simulink model "building_EXAMPLE_v2_r2018b"  (R2018b)
settings: Solver=ode23tb  StartTime=-building.preruntime+8760*3600  StopTime=building.runtime+8760*3600  MaxStep=600  EnableMultiTasking=on
StartFcn:
  | tic
StopFcn:
  | toc
values from neighbouring files (symbols this model uses):
  building = building.add_simulation(1, 'Innsbruck - ERV, 120m3/h, 230 g/h', saveAIB, saveBDB, saveBOUNDARY, saveHVAC, 1)    [work_EXAMPLE_v1.m]
undefined symbols (not defined in the file or in its folder): cp, Dreifach, get_building, p, Qdot_C, Qdot_C_energy, Qdot_H, Qdot_H_energy, Qdot_I_electricity, Qdot_I_electricity_energy, Qdot_I_light, Qdot_I_light_energy, Qdot_I_person, Qdot_I_person_energy, Qdot_S, Qdot_S_energy, Qdot_T_ground, Qdot_T_ground_energy, Qdot_T_neighbour, Qdot_T_neighbour_energy, Qdot_T_opaque, Qdot_T_opaque_energy, Qdot_T_window, Qdot_T_window_energy, Qdot_V_infiltration, Qdot_V_infiltration_energy, Qdot_V_mech, Qdot_V_mech_energy, Qdot_V_window, Qdot_V_window_energy, rho, Tc, Tr, Ts, Wärmeschutzglas, x_CO2, x_H2O, x_VOC
libraries: carnotUIBK x1879, carnot x1
(part 8 of 28)

== system building_EXAMPLE_v2_r2018b/DATALOGGER/AIBz6 ==
  AIB : Inport
  AIB_initialize : carnotUIBK/room_node/EMPTY/AIB_initialize  SystemSampleTime=-1
  Bus Assignment1 : BusAssignment  AssignedSignals=Ts,Tc,Tr,x_H2O,x_CO2,x_VOC,rho,cp,p
  Bus Selector1 : BusSelector  OutputSignals=Ts,Tc,Tr,x_H2O,x_CO2,x_VOC,rho,cp,p
  AIB' : Outport
  wires:
  Bus Selector1/8 -> Bus Assignment1/9  "<cp>"
  Bus Selector1/7 -> Bus Assignment1/8  "<rho>"
  Bus Selector1/6 -> Bus Assignment1/7  "<x_VOC>"
  Bus Selector1/5 -> Bus Assignment1/6  "<x_CO2>"
  Bus Selector1/2 -> Bus Assignment1/3  "<Tc>"
  Bus Selector1/4 -> Bus Assignment1/5  "<x_H2O>"
  Bus Selector1/9 -> Bus Assignment1/10  "<p>"
  Bus Selector1/3 -> Bus Assignment1/4  "<Tr>"
  Bus Selector1/1 -> Bus Assignment1/2  "<Ts>"
  AIB_initialize/1 -> Bus Assignment1/1
  AIB/1 -> Bus Selector1/1
  Bus Assignment1/1 -> AIB'/1

== system building_EXAMPLE_v2_r2018b/DATALOGGER/AIBz7 ==
  AIB : Inport
  AIB_initialize : carnotUIBK/room_node/EMPTY/AIB_initialize  SystemSampleTime=-1
  Bus Assignment1 : BusAssignment  AssignedSignals=Ts,Tc,Tr,x_H2O,x_CO2,x_VOC,rho,cp,p
  Bus Selector1 : BusSelector  OutputSignals=Ts,Tc,Tr,x_H2O,x_CO2,x_VOC,rho,cp,p
  AIB' : Outport
  wires:
  Bus Assignment1/1 -> AIB'/1
  AIB/1 -> Bus Selector1/1
  AIB_initialize/1 -> Bus Assignment1/1
  Bus Selector1/1 -> Bus Assignment1/2  "<Ts>"
  Bus Selector1/3 -> Bus Assignment1/4  "<Tr>"
  Bus Selector1/9 -> Bus Assignment1/10  "<p>"
  Bus Selector1/4 -> Bus Assignment1/5  "<x_H2O>"
  Bus Selector1/2 -> Bus Assignment1/3  "<Tc>"
  Bus Selector1/5 -> Bus Assignment1/6  "<x_CO2>"
  Bus Selector1/6 -> Bus Assignment1/7  "<x_VOC>"
  Bus Selector1/7 -> Bus Assignment1/8  "<rho>"
  Bus Selector1/8 -> Bus Assignment1/9  "<cp>"

== system building_EXAMPLE_v2_r2018b/DATALOGGER/AIBz8 ==
  AIB : Inport
  AIB_initialize : carnotUIBK/room_node/EMPTY/AIB_initialize  SystemSampleTime=-1
  Bus Assignment1 : BusAssignment  AssignedSignals=Ts,Tc,Tr,x_H2O,x_CO2,x_VOC,rho,cp,p
  Bus Selector1 : BusSelector  OutputSignals=Ts,Tc,Tr,x_H2O,x_CO2,x_VOC,rho,cp,p
  AIB' : Outport
  wires:
  Bus Selector1/8 -> Bus Assignment1/9  "<cp>"
  Bus Selector1/7 -> Bus Assignment1/8  "<rho>"
  Bus Selector1/6 -> Bus Assignment1/7  "<x_VOC>"
  Bus Selector1/5 -> Bus Assignment1/6  "<x_CO2>"
  Bus Selector1/2 -> Bus Assignment1/3  "<Tc>"
  Bus Selector1/4 -> Bus Assignment1/5  "<x_H2O>"
  Bus Selector1/9 -> Bus Assignment1/10  "<p>"
  Bus Selector1/3 -> Bus Assignment1/4  "<Tr>"
  Bus Selector1/1 -> Bus Assignment1/2  "<Ts>"
  AIB_initialize/1 -> Bus Assignment1/1
  AIB/1 -> Bus Selector1/1
  Bus Assignment1/1 -> AIB'/1

== system building_EXAMPLE_v2_r2018b/DATALOGGER/AIBz9 ==
  AIB : Inport
  AIB_initialize : carnotUIBK/room_node/EMPTY/AIB_initialize  SystemSampleTime=-1
  Bus Assignment1 : BusAssignment  AssignedSignals=Ts,Tc,Tr,x_H2O,x_CO2,x_VOC,rho,cp,p
  Bus Selector1 : BusSelector  OutputSignals=Ts,Tc,Tr,x_H2O,x_CO2,x_VOC,rho,cp,p
  AIB' : Outport
  wires:
  Bus Assignment1/1 -> AIB'/1
  AIB/1 -> Bus Selector1/1
  AIB_initialize/1 -> Bus Assignment1/1
  Bus Selector1/1 -> Bus Assignment1/2  "<Ts>"
  Bus Selector1/3 -> Bus Assignment1/4  "<Tr>"
  Bus Selector1/9 -> Bus Assignment1/10  "<p>"
  Bus Selector1/4 -> Bus Assignment1/5  "<x_H2O>"
  Bus Selector1/2 -> Bus Assignment1/3  "<Tc>"
  Bus Selector1/5 -> Bus Assignment1/6  "<x_CO2>"
  Bus Selector1/6 -> Bus Assignment1/7  "<x_VOC>"
  Bus Selector1/7 -> Bus Assignment1/8  "<rho>"
  Bus Selector1/8 -> Bus Assignment1/9  "<cp>"

== system building_EXAMPLE_v2_r2018b/DATALOGGER/logger_AIB ==
  AIB : Inport
  Enable : EnablePort
  saveAIB : ToWorkspace  VariableName=saveAIB  SaveFormat=Timeseries  SampleTime=building.get_building().sampletime_1
  wires:
  AIB/1 -> saveAIB/1

== system building_EXAMPLE_v2_r2018b/DATALOGGER/logger_BDB ==
  note: CHANGE BDB TO THE CORRESPONDING ZONE!!!!
  BDB : Inport
  Enable : EnablePort
  Bus Creator : BusCreator  Inputs=2
  Bus Creator1 : BusCreator  Inputs=10
  saveBDB : ToWorkspace  VariableName=saveBDB  SaveFormat=Timeseries  SampleTime=building.get_building().sampletime_1
  z1 : Subsystem
  z10 : Subsystem
  z2 : Subsystem
  z3 : Subsystem
  z4 : Subsystem
  z5 : Subsystem
  z6 : Subsystem
  z7 : Subsystem
  z8 : Subsystem
  z9 : Subsystem
  wires:
  BDB/1 -> Bus Creator/1, z1/1(BDB), z2/1(BDB), z3/1(BDB), z4/1(BDB), z5/1(BDB), z6/1(BDB), z7/1(BDB), z8/1(BDB), z10/1(BDB), z9/1(BDB)  "power"
  Bus Creator/1 -> saveBDB/1
  z1/1(BDBenergy) -> Bus Creator1/1  "z1"
  z4/1(BDBenergy) -> Bus Creator1/4  "z4"
  z3/1(BDBenergy) -> Bus Creator1/3  "z3"
  z2/1(BDBenergy) -> Bus Creator1/2  "z2"
  z10/1(BDBenergy) -> Bus Creator1/10  "z10"
  z9/1(BDBenergy) -> Bus Creator1/9  "z9"
  z8/1(BDBenergy) -> Bus Creator1/8  "z8"
  z7/1(BDBenergy) -> Bus Creator1/7  "z7"
  z6/1(BDBenergy) -> Bus Creator1/6  "z6"
  z5/1(BDBenergy) -> Bus Creator1/5  "z5"
  Bus Creator1/1 -> Bus Creator/2  "energy"

== system building_EXAMPLE_v2_r2018b/DATALOGGER/logger_BOUNDARY ==
  BOUNDARY : Inport
  Enable : EnablePort
  Bus Creator : BusCreator  Inputs=2
  Bus Creator1 : BusCreator  Inputs=4
  Bus Selector : BusSelector  OutputSignals=WDB.Solar_Radiation_beam_normal,WDB.Solar_Radiation_diffuse_horizontal,WDB.Solar_Radiation_direct_surface,WDB.Solar_Radiation_diffuse_surface  OutputAsBus=on
  Demux : Demux
  Integrator : Integrator
  Ws->kWh : Gain  Gain=1/3600/1000
  saveBOUNDARY : ToWorkspace  VariableName=saveBOUNDARY  SaveFormat=Timeseries  SampleTime=building.get_building().sampletime_1
  wires:
  BOUNDARY/1 -> Bus Selector/1, Bus Creator/1  "power"
  Bus Creator/1 -> saveBOUNDARY/1
  Bus Selector/1 -> Integrator/1
  Integrator/1 -> Ws->kWh/1
  Demux/1 -> Bus Creator1/1  "Solar_Radiation_beam_normal_Energy"
  Demux/2 -> Bus Creator1/2  "Solar_Radiation_diffuse_horizontal_Energy"
  Demux/4 -> Bus Creator1/4  "Solar_Radiation_diffuse_surface_Energy"
  Demux/3 -> Bus Creator1/3  "Solar_Radiation_direct_surface_Energy"
  Bus Creator1/1 -> Bus Creator/2  "energy"
  Ws->kWh/1 -> Demux/1

== system building_EXAMPLE_v2_r2018b/DATALOGGER/logger_HVAC ==
  HVAC : Inport
  Enable : EnablePort
  saveHVAC : ToWorkspace  VariableName=saveHVAC  SaveFormat=Timeseries  SampleTime=building.get_building().sampletime_1
  wires:
  HVAC/1 -> saveHVAC/1

== system building_EXAMPLE_v2_r2018b/DATALOGGER/z1 ==
  BDB : Inport
  BDB_initialize : carnotUIBK/room_node/EMPTY/BDB_initialize  SystemSampleTime=-1
  Bus Assignment : BusAssignment  AssignedSignals=Qdot_T_opaque,Qdot_T_ground,Qdot_T_neighbour,Qdot_T_window,Qdot_V_mech,Qdot_V_window,Qdot_V_infiltration,Qdot_S,Qdot_I_person,Qdot_I_light,Qdot_I_electricity,Qdot_H,Qdot_C
  Bus Selector1 : BusSelector  OutputSignals=Qdot_T_opaque,Qdot_T_ground,Qdot_T_neighbour,Qdot_T_window,Qdot_V_mech,Qdot_V_window,Qdot_V_infiltration,Qdot_S,Qdot_I_person,Qdot_I_light,Qdot_I_electricity,Qdot_H,Qdot_C
  BDB' : Outport
  wires:
  BDB/1 -> Bus Selector1/1
  Bus Assignment/1 -> BDB'/1
  BDB_initialize/1 -> Bus Assignment/1
  Bus Selector1/1 -> Bus Assignment/2  "<Qdot_T_opaque>"
  Bus Selector1/13 -> Bus Assignment/14  "<Qdot_C>"
  Bus Selector1/12 -> Bus Assignment/13  "<Qdot_H>"
  Bus Selector1/11 -> Bus Assignment/12  "<Qdot_I_electricity>"
  Bus Selector1/10 -> Bus Assignment/11  "<Qdot_I_light>"
  Bus Selector1/9 -> Bus Assignment/10  "<Qdot_I_person>"
  Bus Selector1/8 -> Bus Assignment/9  "<Qdot_S>"
  Bus Selector1/7 -> Bus Assignment/8  "<Qdot_V_infiltration>"
  Bus Selector1/6 -> Bus Assignment/7  "<Qdot_V_window>"
  Bus Selector1/5 -> Bus Assignment/6  "<Qdot_V_mech>"
  Bus Selector1/4 -> Bus Assignment/5  "<Qdot_T_window>"
  Bus Selector1/3 -> Bus Assignment/4  "<Qdot_T_neighbour>"
  Bus Selector1/2 -> Bus Assignment/3  "<Qdot_T_ground>"

== system building_EXAMPLE_v2_r2018b/DATALOGGER/z10 ==
  BDB : Inport
  BDB_initialize : carnotUIBK/room_node/EMPTY/BDB_initialize  SystemSampleTime=-1
  Bus Assignment : BusAssignment  AssignedSignals=Qdot_T_opaque,Qdot_T_ground,Qdot_T_neighbour,Qdot_T_window,Qdot_V_mech,Qdot_V_window,Qdot_V_infiltration,Qdot_S,Qdot_I_person,Qdot_I_light,Qdot_I_electricity,Qdot_H,Qdot_C
  Bus Selector1 : BusSelector  OutputSignals=Qdot_T_opaque,Qdot_T_ground,Qdot_T_neighbour,Qdot_T_window,Qdot_V_mech,Qdot_V_window,Qdot_V_infiltration,Qdot_S,Qdot_I_person,Qdot_I_light,Qdot_I_electricity,Qdot_H,Qdot_C
  BDB' : Outport
  wires:
  Bus Selector1/2 -> Bus Assignment/3  "<Qdot_T_ground>"
  Bus Selector1/3 -> Bus Assignment/4  "<Qdot_T_neighbour>"
  Bus Selector1/4 -> Bus Assignment/5  "<Qdot_T_window>"
  Bus Selector1/5 -> Bus Assignment/6  "<Qdot_V_mech>"
  Bus Selector1/6 -> Bus Assignment/7  "<Qdot_V_window>"
  Bus Selector1/7 -> Bus Assignment/8  "<Qdot_V_infiltration>"
  Bus Selector1/8 -> Bus Assignment/9  "<Qdot_S>"
  Bus Selector1/9 -> Bus Assignment/10  "<Qdot_I_person>"
  Bus Selector1/10 -> Bus Assignment/11  "<Qdot_I_light>"
  Bus Selector1/11 -> Bus Assignment/12  "<Qdot_I_electricity>"
  Bus Selector1/12 -> Bus Assignment/13  "<Qdot_H>"
  Bus Selector1/13 -> Bus Assignment/14  "<Qdot_C>"
  Bus Selector1/1 -> Bus Assignment/2  "<Qdot_T_opaque>"
  BDB_initialize/1 -> Bus Assignment/1
  Bus Assignment/1 -> BDB'/1
  BDB/1 -> Bus Selector1/1

== system building_EXAMPLE_v2_r2018b/DATALOGGER/z2 ==
  BDB : Inport
  BDB_initialize : carnotUIBK/room_node/EMPTY/BDB_initialize  SystemSampleTime=-1
  Bus Assignment : BusAssignment  AssignedSignals=Qdot_T_opaque,Qdot_T_ground,Qdot_T_neighbour,Qdot_T_window,Qdot_V_mech,Qdot_V_window,Qdot_V_infiltration,Qdot_S,Qdot_I_person,Qdot_I_light,Qdot_I_electricity,Qdot_H,Qdot_C
  Bus Selector1 : BusSelector  OutputSignals=Qdot_T_opaque,Qdot_T_ground,Qdot_T_neighbour,Qdot_T_window,Qdot_V_mech,Qdot_V_window,Qdot_V_infiltration,Qdot_S,Qdot_I_person,Qdot_I_light,Qdot_I_electricity,Qdot_H,Qdot_C
  BDB' : Outport
  wires:
  Bus Selector1/2 -> Bus Assignment/3  "<Qdot_T_ground>"
  Bus Selector1/3 -> Bus Assignment/4  "<Qdot_T_neighbour>"
  Bus Selector1/4 -> Bus Assignment/5  "<Qdot_T_window>"
  Bus Selector1/5 -> Bus Assignment/6  "<Qdot_V_mech>"
  Bus Selector1/6 -> Bus Assignment/7  "<Qdot_V_window>"
  Bus Selector1/7 -> Bus Assignment/8  "<Qdot_V_infiltration>"
  Bus Selector1/8 -> Bus Assignment/9  "<Qdot_S>"
  Bus Selector1/9 -> Bus Assignment/10  "<Qdot_I_person>"
  Bus Selector1/10 -> Bus Assignment/11  "<Qdot_I_light>"
  Bus Selector1/11 -> Bus Assignment/12  "<Qdot_I_electricity>"
  Bus Selector1/12 -> Bus Assignment/13  "<Qdot_H>"
  Bus Selector1/13 -> Bus Assignment/14  "<Qdot_C>"
  Bus Selector1/1 -> Bus Assignment/2  "<Qdot_T_opaque>"
  BDB_initialize/1 -> Bus Assignment/1
  Bus Assignment/1 -> BDB'/1
  BDB/1 -> Bus Selector1/1

== system building_EXAMPLE_v2_r2018b/DATALOGGER/z3 ==
  BDB : Inport
  BDB_initialize : carnotUIBK/room_node/EMPTY/BDB_initialize  SystemSampleTime=-1
  Bus Assignment : BusAssignment  AssignedSignals=Qdot_T_opaque,Qdot_T_ground,Qdot_T_neighbour,Qdot_T_window,Qdot_V_mech,Qdot_V_window,Qdot_V_infiltration,Qdot_S,Qdot_I_person,Qdot_I_light,Qdot_I_electricity,Qdot_H,Qdot_C
  Bus Selector1 : BusSelector  OutputSignals=Qdot_T_opaque,Qdot_T_ground,Qdot_T_neighbour,Qdot_T_window,Qdot_V_mech,Qdot_V_window,Qdot_V_infiltration,Qdot_S,Qdot_I_person,Qdot_I_light,Qdot_I_electricity,Qdot_H,Qdot_C
  BDB' : Outport
  wires:
  BDB/1 -> Bus Selector1/1
  Bus Assignment/1 -> BDB'/1
  BDB_initialize/1 -> Bus Assignment/1
  Bus Selector1/1 -> Bus Assignment/2  "<Qdot_T_opaque>"
  Bus Selector1/13 -> Bus Assignment/14  "<Qdot_C>"
  Bus Selector1/12 -> Bus Assignment/13  "<Qdot_H>"
  Bus Selector1/11 -> Bus Assignment/12  "<Qdot_I_electricity>"
  Bus Selector1/10 -> Bus Assignment/11  "<Qdot_I_light>"
  Bus Selector1/9 -> Bus Assignment/10  "<Qdot_I_person>"
  Bus Selector1/8 -> Bus Assignment/9  "<Qdot_S>"
  Bus Selector1/7 -> Bus Assignment/8  "<Qdot_V_infiltration>"
  Bus Selector1/6 -> Bus Assignment/7  "<Qdot_V_window>"
  Bus Selector1/5 -> Bus Assignment/6  "<Qdot_V_mech>"
  Bus Selector1/4 -> Bus Assignment/5  "<Qdot_T_window>"
  Bus Selector1/3 -> Bus Assignment/4  "<Qdot_T_neighbour>"
  Bus Selector1/2 -> Bus Assignment/3  "<Qdot_T_ground>"

== system building_EXAMPLE_v2_r2018b/DATALOGGER/z4 ==
  BDB : Inport
  BDB_initialize : carnotUIBK/room_node/EMPTY/BDB_initialize  SystemSampleTime=-1
  Bus Assignment : BusAssignment  AssignedSignals=Qdot_T_opaque,Qdot_T_ground,Qdot_T_neighbour,Qdot_T_window,Qdot_V_mech,Qdot_V_window,Qdot_V_infiltration,Qdot_S,Qdot_I_person,Qdot_I_light,Qdot_I_electricity,Qdot_H,Qdot_C
  Bus Selector1 : BusSelector  OutputSignals=Qdot_T_opaque,Qdot_T_ground,Qdot_T_neighbour,Qdot_T_window,Qdot_V_mech,Qdot_V_window,Qdot_V_infiltration,Qdot_S,Qdot_I_person,Qdot_I_light,Qdot_I_electricity,Qdot_H,Qdot_C
  BDB' : Outport
  wires:
  Bus Selector1/2 -> Bus Assignment/3  "<Qdot_T_ground>"
  Bus Selector1/3 -> Bus Assignment/4  "<Qdot_T_neighbour>"
  Bus Selector1/4 -> Bus Assignment/5  "<Qdot_T_window>"
  Bus Selector1/5 -> Bus Assignment/6  "<Qdot_V_mech>"
  Bus Selector1/6 -> Bus Assignment/7  "<Qdot_V_window>"
  Bus Selector1/7 -> Bus Assignment/8  "<Qdot_V_infiltration>"
  Bus Selector1/8 -> Bus Assignment/9  "<Qdot_S>"
  Bus Selector1/9 -> Bus Assignment/10  "<Qdot_I_person>"
  Bus Selector1/10 -> Bus Assignment/11  "<Qdot_I_light>"
  Bus Selector1/11 -> Bus Assignment/12  "<Qdot_I_electricity>"
  Bus Selector1/12 -> Bus Assignment/13  "<Qdot_H>"
  Bus Selector1/13 -> Bus Assignment/14  "<Qdot_C>"
  Bus Selector1/1 -> Bus Assignment/2  "<Qdot_T_opaque>"
  BDB_initialize/1 -> Bus Assignment/1
  Bus Assignment/1 -> BDB'/1
  BDB/1 -> Bus Selector1/1

== system building_EXAMPLE_v2_r2018b/DATALOGGER/z5 ==
  BDB : Inport
  BDB_initialize : carnotUIBK/room_node/EMPTY/BDB_initialize  SystemSampleTime=-1
  Bus Assignment : BusAssignment  AssignedSignals=Qdot_T_opaque,Qdot_T_ground,Qdot_T_neighbour,Qdot_T_window,Qdot_V_mech,Qdot_V_window,Qdot_V_infiltration,Qdot_S,Qdot_I_person,Qdot_I_light,Qdot_I_electricity,Qdot_H,Qdot_C
  Bus Selector1 : BusSelector  OutputSignals=Qdot_T_opaque,Qdot_T_ground,Qdot_T_neighbour,Qdot_T_window,Qdot_V_mech,Qdot_V_window,Qdot_V_infiltration,Qdot_S,Qdot_I_person,Qdot_I_light,Qdot_I_electricity,Qdot_H,Qdot_C
  BDB' : Outport
  wires:
  BDB/1 -> Bus Selector1/1
  Bus Assignment/1 -> BDB'/1
  BDB_initialize/1 -> Bus Assignment/1
  Bus Selector1/1 -> Bus Assignment/2  "<Qdot_T_opaque>"
  Bus Selector1/13 -> Bus Assignment/14  "<Qdot_C>"
  Bus Selector1/12 -> Bus Assignment/13  "<Qdot_H>"
  Bus Selector1/11 -> Bus Assignment/12  "<Qdot_I_electricity>"
  Bus Selector1/10 -> Bus Assignment/11  "<Qdot_I_light>"
  Bus Selector1/9 -> Bus Assignment/10  "<Qdot_I_person>"
  Bus Selector1/8 -> Bus Assignment/9  "<Qdot_S>"
  Bus Selector1/7 -> Bus Assignment/8  "<Qdot_V_infiltration>"
  Bus Selector1/6 -> Bus Assignment/7  "<Qdot_V_window>"
  Bus Selector1/5 -> Bus Assignment/6  "<Qdot_V_mech>"
  Bus Selector1/4 -> Bus Assignment/5  "<Qdot_T_window>"
  Bus Selector1/3 -> Bus Assignment/4  "<Qdot_T_neighbour>"
  Bus Selector1/2 -> Bus Assignment/3  "<Qdot_T_ground>"

== system building_EXAMPLE_v2_r2018b/DATALOGGER/z6 ==
  BDB : Inport
  BDB_initialize : carnotUIBK/room_node/EMPTY/BDB_initialize  SystemSampleTime=-1
  Bus Assignment : BusAssignment  AssignedSignals=Qdot_T_opaque,Qdot_T_ground,Qdot_T_neighbour,Qdot_T_window,Qdot_V_mech,Qdot_V_window,Qdot_V_infiltration,Qdot_S,Qdot_I_person,Qdot_I_light,Qdot_I_electricity,Qdot_H,Qdot_C
  Bus Selector1 : BusSelector  OutputSignals=Qdot_T_opaque,Qdot_T_ground,Qdot_T_neighbour,Qdot_T_window,Qdot_V_mech,Qdot_V_window,Qdot_V_infiltration,Qdot_S,Qdot_I_person,Qdot_I_light,Qdot_I_electricity,Qdot_H,Qdot_C
  BDB' : Outport
  wires:
  Bus Selector1/2 -> Bus Assignment/3  "<Qdot_T_ground>"
  Bus Selector1/3 -> Bus Assignment/4  "<Qdot_T_neighbour>"
  Bus Selector1/4 -> Bus Assignment/5  "<Qdot_T_window>"
  Bus Selector1/5 -> Bus Assignment/6  "<Qdot_V_mech>"
  Bus Selector1/6 -> Bus Assignment/7  "<Qdot_V_window>"
  Bus Selector1/7 -> Bus Assignment/8  "<Qdot_V_infiltration>"
  Bus Selector1/8 -> Bus Assignment/9  "<Qdot_S>"
  Bus Selector1/9 -> Bus Assignment/10  "<Qdot_I_person>"
  Bus Selector1/10 -> Bus Assignment/11  "<Qdot_I_light>"
  Bus Selector1/11 -> Bus Assignment/12  "<Qdot_I_electricity>"
  Bus Selector1/12 -> Bus Assignment/13  "<Qdot_H>"
  Bus Selector1/13 -> Bus Assignment/14  "<Qdot_C>"
  Bus Selector1/1 -> Bus Assignment/2  "<Qdot_T_opaque>"
  BDB_initialize/1 -> Bus Assignment/1
  Bus Assignment/1 -> BDB'/1
  BDB/1 -> Bus Selector1/1

== system building_EXAMPLE_v2_r2018b/DATALOGGER/z7 ==
  BDB : Inport
  BDB_initialize : carnotUIBK/room_node/EMPTY/BDB_initialize  SystemSampleTime=-1
  Bus Assignment : BusAssignment  AssignedSignals=Qdot_T_opaque,Qdot_T_ground,Qdot_T_neighbour,Qdot_T_window,Qdot_V_mech,Qdot_V_window,Qdot_V_infiltration,Qdot_S,Qdot_I_person,Qdot_I_light,Qdot_I_electricity,Qdot_H,Qdot_C
  Bus Selector1 : BusSelector  OutputSignals=Qdot_T_opaque,Qdot_T_ground,Qdot_T_neighbour,Qdot_T_window,Qdot_V_mech,Qdot_V_window,Qdot_V_infiltration,Qdot_S,Qdot_I_person,Qdot_I_light,Qdot_I_electricity,Qdot_H,Qdot_C
  BDB' : Outport
  wires:
  BDB/1 -> Bus Selector1/1
  Bus Assignment/1 -> BDB'/1
  BDB_initialize/1 -> Bus Assignment/1
  Bus Selector1/1 -> Bus Assignment/2  "<Qdot_T_opaque>"
  Bus Selector1/13 -> Bus Assignment/14  "<Qdot_C>"
  Bus Selector1/12 -> Bus Assignment/13  "<Qdot_H>"
  Bus Selector1/11 -> Bus Assignment/12  "<Qdot_I_electricity>"
  Bus Selector1/10 -> Bus Assignment/11  "<Qdot_I_light>"
  Bus Selector1/9 -> Bus Assignment/10  "<Qdot_I_person>"
  Bus Selector1/8 -> Bus Assignment/9  "<Qdot_S>"
  Bus Selector1/7 -> Bus Assignment/8  "<Qdot_V_infiltration>"
  Bus Selector1/6 -> Bus Assignment/7  "<Qdot_V_window>"
  Bus Selector1/5 -> Bus Assignment/6  "<Qdot_V_mech>"
  Bus Selector1/4 -> Bus Assignment/5  "<Qdot_T_window>"
  Bus Selector1/3 -> Bus Assignment/4  "<Qdot_T_neighbour>"
  Bus Selector1/2 -> Bus Assignment/3  "<Qdot_T_ground>"

== system building_EXAMPLE_v2_r2018b/DATALOGGER/z8 ==
  BDB : Inport
  BDB_initialize : carnotUIBK/room_node/EMPTY/BDB_initialize  SystemSampleTime=-1
  Bus Assignment : BusAssignment  AssignedSignals=Qdot_T_opaque,Qdot_T_ground,Qdot_T_neighbour,Qdot_T_window,Qdot_V_mech,Qdot_V_window,Qdot_V_infiltration,Qdot_S,Qdot_I_person,Qdot_I_light,Qdot_I_electricity,Qdot_H,Qdot_C
  Bus Selector1 : BusSelector  OutputSignals=Qdot_T_opaque,Qdot_T_ground,Qdot_T_neighbour,Qdot_T_window,Qdot_V_mech,Qdot_V_window,Qdot_V_infiltration,Qdot_S,Qdot_I_person,Qdot_I_light,Qdot_I_electricity,Qdot_H,Qdot_C
  BDB' : Outport
  wires:
  Bus Selector1/2 -> Bus Assignment/3  "<Qdot_T_ground>"
  Bus Selector1/3 -> Bus Assignment/4  "<Qdot_T_neighbour>"
  Bus Selector1/4 -> Bus Assignment/5  "<Qdot_T_window>"
  Bus Selector1/5 -> Bus Assignment/6  "<Qdot_V_mech>"
  Bus Selector1/6 -> Bus Assignment/7  "<Qdot_V_window>"
  Bus Selector1/7 -> Bus Assignment/8  "<Qdot_V_infiltration>"
  Bus Selector1/8 -> Bus Assignment/9  "<Qdot_S>"
  Bus Selector1/9 -> Bus Assignment/10  "<Qdot_I_person>"
  Bus Selector1/10 -> Bus Assignment/11  "<Qdot_I_light>"
  Bus Selector1/11 -> Bus Assignment/12  "<Qdot_I_electricity>"
  Bus Selector1/12 -> Bus Assignment/13  "<Qdot_H>"
  Bus Selector1/13 -> Bus Assignment/14  "<Qdot_C>"
  Bus Selector1/1 -> Bus Assignment/2  "<Qdot_T_opaque>"
  BDB_initialize/1 -> Bus Assignment/1
  Bus Assignment/1 -> BDB'/1
  BDB/1 -> Bus Selector1/1

== system building_EXAMPLE_v2_r2018b/DATALOGGER/z9 ==
  BDB : Inport
  BDB_initialize : carnotUIBK/room_node/EMPTY/BDB_initialize  SystemSampleTime=-1
  Bus Assignment : BusAssignment  AssignedSignals=Qdot_T_opaque,Qdot_T_ground,Qdot_T_neighbour,Qdot_T_window,Qdot_V_mech,Qdot_V_window,Qdot_V_infiltration,Qdot_S,Qdot_I_person,Qdot_I_light,Qdot_I_electricity,Qdot_H,Qdot_C
  Bus Selector1 : BusSelector  OutputSignals=Qdot_T_opaque,Qdot_T_ground,Qdot_T_neighbour,Qdot_T_window,Qdot_V_mech,Qdot_V_window,Qdot_V_infiltration,Qdot_S,Qdot_I_person,Qdot_I_light,Qdot_I_electricity,Qdot_H,Qdot_C
  BDB' : Outport
  wires:
  BDB/1 -> Bus Selector1/1
  Bus Assignment/1 -> BDB'/1
  BDB_initialize/1 -> Bus Assignment/1
  Bus Selector1/1 -> Bus Assignment/2  "<Qdot_T_opaque>"
  Bus Selector1/13 -> Bus Assignment/14  "<Qdot_C>"
  Bus Selector1/12 -> Bus Assignment/13  "<Qdot_H>"
  Bus Selector1/11 -> Bus Assignment/12  "<Qdot_I_electricity>"
  Bus Selector1/10 -> Bus Assignment/11  "<Qdot_I_light>"
  Bus Selector1/9 -> Bus Assignment/10  "<Qdot_I_person>"
  Bus Selector1/8 -> Bus Assignment/9  "<Qdot_S>"
  Bus Selector1/7 -> Bus Assignment/8  "<Qdot_V_infiltration>"
  Bus Selector1/6 -> Bus Assignment/7  "<Qdot_V_window>"
  Bus Selector1/5 -> Bus Assignment/6  "<Qdot_V_mech>"
  Bus Selector1/4 -> Bus Assignment/5  "<Qdot_T_window>"
  Bus Selector1/3 -> Bus Assignment/4  "<Qdot_T_neighbour>"
  Bus Selector1/2 -> Bus Assignment/3  "<Qdot_T_ground>"

== system building_EXAMPLE_v2_r2018b/BUILDING/INTERSECTION_1_10/airexchange_1 ==
  AIB1 : Inport
  AIB2 : Inport  Port=2
  control : Inport  Port=3
  EMPTY : carnotUIBK/airexchange_intersection/EMPTY  VariantControl=(default)
  airexchange_empiric : carnotUIBK/airexchange_intersection/airexchange_empiric  VariantControl=V_i_1_10_inf1_m0
  airexchange_powerlaw : carnotUIBK/airexchange_intersection/airexchange_powerlaw  VariantControl=V_i_1_10_inf1_m1
  "[S1]" : Outport
  "[S2]" : Outport  Port=2

== system building_EXAMPLE_v2_r2018b/BUILDING/INTERSECTION_1_10/airexchange_2 ==
  AIB1 : Inport
  AIB2 : Inport  Port=2
  control : Inport  Port=3
  EMPTY : carnotUIBK/airexchange_intersection/EMPTY  VariantControl=(default)
  airexchange_empiric : carnotUIBK/airexchange_intersection/airexchange_empiric  VariantControl=V_i_1_10_inf2_m0
  airexchange_powerlaw : carnotUIBK/airexchange_intersection/airexchange_powerlaw  VariantControl=V_i_1_10_inf2_m1
  "[S1]" : Outport
  "[S2]" : Outport  Port=2

== system building_EXAMPLE_v2_r2018b/BUILDING/INTERSECTION_1_10/airexchange_3 ==
  AIB1 : Inport
  AIB2 : Inport  Port=2
  control : Inport  Port=3
  EMPTY : carnotUIBK/airexchange_intersection/EMPTY  VariantControl=(default)
  airexchange_empiric : carnotUIBK/airexchange_intersection/airexchange_empiric  VariantControl=V_i_1_10_inf3_m0
  airexchange_powerlaw : carnotUIBK/airexchange_intersection/airexchange_powerlaw  VariantControl=V_i_1_10_inf3_m1
  "[S1]" : Outport
  "[S2]" : Outport  Port=2

== system building_EXAMPLE_v2_r2018b/BUILDING/INTERSECTION_1_10/wall_1 ==
  AIB1 : Inport
  AIB2 : Inport  Port=2
  Qdot_sol1 : Inport  Port=3
  Qdot_sol2 : Inport  Port=4
  EMPTY : carnotUIBK/wall_intersection/EMPTY  VariantControl=(default)
  R-C model : carnotUIBK/wall_intersection/R-C model  VariantControl=V_i_1_10_w1_m1  t0=z.t_ini  d=fliplr(const.parameter.xmesh_beu)  cond=fliplr(const.parameter.lambda)  cwall=fliplr(const.parameter.cp)  rho=fliplr(const.parameter.rho)  reflectground=0.2  abs_emiss=[const.absorption_2 const.emission_2 const.emission_1]  tau=const.parameter.tau  dactive=const.parameter.d_active
      link override alpha_i1/alpha_i_down: VariantControl=V_i_1_10_w1_hti2
      link override alpha_i1/alpha_i_horizontal: VariantControl=V_i_1_10_w1_hti0
      link override alpha_i1/alpha_i_up: VariantControl=V_i_1_10_w1_hti1
      link override alpha_i2/alpha_i_down: VariantControl=V_i_1_10_w1_hti2
      link override alpha_i2/alpha_i_horizontal: VariantControl=V_i_1_10_w1_hti0
      link override alpha_i2/alpha_i_up: VariantControl=V_i_1_10_w1_hti1
  UA : carnotUIBK/wall_intersection/UA  VariantControl=V_i_1_10_w1_m0  U=const.parameter.U
      link override Rsi/down: VariantControl=V_i_1_10_w1_hti2
      link override Rsi/horizontal: VariantControl=V_i_1_10_w1_hti0
      link override Rsi/up: VariantControl=V_i_1_10_w1_hti1
  hygrothermal model : carnotUIBK/wall_intersection/hygrothermal model  VariantControl=V_i_1_10_w1_m2  t0=z.t_ini  reflectground=0.2  abs_emiss=[const.absorption_2 const.emission_2 const.emission_1]  xmesh=const.parameter.xmesh_hygro  X=const.parameter.X  d=const.parameter.d  lambda=const.parameter.lambda_hygro  rho=const.parameter.rho_hygro  cp=const.parameter.cp_hygro  mu=const.parameter.mu  ufs=const.parameter.ufs  FSF_u=const.parameter.FSF_u  FSF_phi=const.parameter.FSF_phi  FSF_dudphi=const.parameter.FSF_dudphi  FSF_k=const.parameter.FSF_k  K_kleff=const.parameter.K_kleff  K_u=const.parameter.K_u  K_kl=const.parameter.K_kl  FSF_length=const.parameter.FSF_length  K_length=const.parameter.K_length  T_ini=const.parameter.T_ini_hygro  Phi_ini=const.parameter.Phi_ini_hygro  T_source=const.parameter.T_source  Phi_source=const.parameter.Phi_source  Tdactive=const.parameter.T_dactive  Phidactive=const.parameter.Phi_dactive
      link override alpha_i1/alpha_i_down: VariantControl=V_i_1_10_w1_hti2
      link override alpha_i1/alpha_i_horizontal: VariantControl=V_i_1_10_w1_hti0
      link override alpha_i1/alpha_i_up: VariantControl=V_i_1_10_w1_hti1
      link override alpha_i2/alpha_i_down: VariantControl=V_i_1_10_w1_hti2
      link override alpha_i2/alpha_i_horizontal: VariantControl=V_i_1_10_w1_hti0
      link override alpha_i2/alpha_i_up: VariantControl=V_i_1_10_w1_hti1
  "[S1]" : Outport
  "[S2]" : Outport  Port=2

== system building_EXAMPLE_v2_r2018b/BUILDING/INTERSECTION_1_10/wall_2 ==
  AIB1 : Inport
  AIB2 : Inport  Port=2
  Qdot_sol1 : Inport  Port=3
  Qdot_sol2 : Inport  Port=4
  EMPTY : carnotUIBK/wall_intersection/EMPTY  VariantControl=(default)
  R-C model : carnotUIBK/wall_intersection/R-C model  VariantControl=V_i_1_10_w2_m1  t0=z.t_ini  d=fliplr(const.parameter.xmesh_beu)  cond=fliplr(const.parameter.lambda)  cwall=fliplr(const.parameter.cp)  rho=fliplr(const.parameter.rho)  reflectground=0.2  abs_emiss=[const.absorption_2 const.emission_2 const.emission_1]  tau=const.parameter.tau  dactive=const.parameter.d_active
      link override alpha_i1/alpha_i_down: VariantControl=V_i_1_10_w2_hti2
      link override alpha_i1/alpha_i_horizontal: VariantControl=V_i_1_10_w2_hti0
      link override alpha_i1/alpha_i_up: VariantControl=V_i_1_10_w2_hti1
      link override alpha_i2/alpha_i_down: VariantControl=V_i_1_10_w2_hti2
      link override alpha_i2/alpha_i_horizontal: VariantControl=V_i_1_10_w2_hti0
      link override alpha_i2/alpha_i_up: VariantControl=V_i_1_10_w2_hti1
  UA : carnotUIBK/wall_intersection/UA  VariantControl=V_i_1_10_w2_m0  U=const.parameter.U
      link override Rsi/down: VariantControl=V_i_1_10_w2_hti2
      link override Rsi/horizontal: VariantControl=V_i_1_10_w2_hti0
      link override Rsi/up: VariantControl=V_i_1_10_w2_hti1
  hygrothermal model : carnotUIBK/wall_intersection/hygrothermal model  VariantControl=V_i_1_10_w2_m2  t0=z.t_ini  reflectground=0.2  abs_emiss=[const.absorption_2 const.emission_2 const.emission_1]  xmesh=const.parameter.xmesh_hygro  X=const.parameter.X  d=const.parameter.d  lambda=const.parameter.lambda_hygro  rho=const.parameter.rho_hygro  cp=const.parameter.cp_hygro  mu=const.parameter.mu  ufs=const.parameter.ufs  FSF_u=const.parameter.FSF_u  FSF_phi=const.parameter.FSF_phi  FSF_dudphi=const.parameter.FSF_dudphi  FSF_k=const.parameter.FSF_k  K_kleff=const.parameter.K_kleff  K_u=const.parameter.K_u  K_kl=const.parameter.K_kl  FSF_length=const.parameter.FSF_length  K_length=const.parameter.K_length  T_ini=const.parameter.T_ini_hygro  Phi_ini=const.parameter.Phi_ini_hygro  T_source=const.parameter.T_source  Phi_source=const.parameter.Phi_source  Tdactive=const.parameter.T_dactive  Phidactive=const.parameter.Phi_dactive
      link override alpha_i1/alpha_i_down: VariantControl=V_i_1_10_w2_hti2
      link override alpha_i1/alpha_i_horizontal: VariantControl=V_i_1_10_w2_hti0
      link override alpha_i1/alpha_i_up: VariantControl=V_i_1_10_w2_hti1
      link override alpha_i2/alpha_i_down: VariantControl=V_i_1_10_w2_hti2
      link override alpha_i2/alpha_i_horizontal: VariantControl=V_i_1_10_w2_hti0
      link override alpha_i2/alpha_i_up: VariantControl=V_i_1_10_w2_hti1
  "[S1]" : Outport
  "[S2]" : Outport  Port=2

== system building_EXAMPLE_v2_r2018b/BUILDING/INTERSECTION_1_10/wall_3 ==
  AIB1 : Inport
  AIB2 : Inport  Port=2
  Qdot_sol1 : Inport  Port=3
  Qdot_sol2 : Inport  Port=4
  EMPTY : carnotUIBK/wall_intersection/EMPTY  VariantControl=(default)
  R-C model : carnotUIBK/wall_intersection/R-C model  VariantControl=V_i_1_10_w3_m1  t0=z.t_ini  d=fliplr(const.parameter.xmesh_beu)  cond=fliplr(const.parameter.lambda)  cwall=fliplr(const.parameter.cp)  rho=fliplr(const.parameter.rho)  reflectground=0.2  abs_emiss=[const.absorption_2 const.emission_2 const.emission_1]  tau=const.parameter.tau  dactive=const.parameter.d_active
      link override alpha_i1/alpha_i_down: VariantControl=V_i_1_10_w3_hti2
      link override alpha_i1/alpha_i_horizontal: VariantControl=V_i_1_10_w3_hti0
      link override alpha_i1/alpha_i_up: VariantControl=V_i_1_10_w3_hti1
      link override alpha_i2/alpha_i_down: VariantControl=V_i_1_10_w3_hti2
      link override alpha_i2/alpha_i_horizontal: VariantControl=V_i_1_10_w3_hti0
      link override alpha_i2/alpha_i_up: VariantControl=V_i_1_10_w3_hti1
  UA : carnotUIBK/wall_intersection/UA  VariantControl=V_i_1_10_w3_m0  U=const.parameter.U
      link override Rsi/down: VariantControl=V_i_1_10_w3_hti2
      link override Rsi/horizontal: VariantControl=V_i_1_10_w3_hti0
      link override Rsi/up: VariantControl=V_i_1_10_w3_hti1
  hygrothermal model : carnotUIBK/wall_intersection/hygrothermal model  VariantControl=V_i_1_10_w3_m2  t0=z.t_ini  reflectground=0.2  abs_emiss=[const.absorption_2 const.emission_2 const.emission_1]  xmesh=const.parameter.xmesh_hygro  X=const.parameter.X  d=const.parameter.d  lambda=const.parameter.lambda_hygro  rho=const.parameter.rho_hygro  cp=const.parameter.cp_hygro  mu=const.parameter.mu  ufs=const.parameter.ufs  FSF_u=const.parameter.FSF_u  FSF_phi=const.parameter.FSF_phi  FSF_dudphi=const.parameter.FSF_dudphi  FSF_k=const.parameter.FSF_k  K_kleff=const.parameter.K_kleff  K_u=const.parameter.K_u  K_kl=const.parameter.K_kl  FSF_length=const.parameter.FSF_length  K_length=const.parameter.K_length  T_ini=const.parameter.T_ini_hygro  Phi_ini=const.parameter.Phi_ini_hygro  T_source=const.parameter.T_source  Phi_source=const.parameter.Phi_source  Tdactive=const.parameter.T_dactive  Phidactive=const.parameter.Phi_dactive
      link override alpha_i1/alpha_i_down: VariantControl=V_i_1_10_w3_hti2
      link override alpha_i1/alpha_i_horizontal: VariantControl=V_i_1_10_w3_hti0
      link override alpha_i1/alpha_i_up: VariantControl=V_i_1_10_w3_hti1
      link override alpha_i2/alpha_i_down: VariantControl=V_i_1_10_w3_hti2
      link override alpha_i2/alpha_i_horizontal: VariantControl=V_i_1_10_w3_hti0
      link override alpha_i2/alpha_i_up: VariantControl=V_i_1_10_w3_hti1
  "[S1]" : Outport
  "[S2]" : Outport  Port=2

== system building_EXAMPLE_v2_r2018b/BUILDING/INTERSECTION_1_2/airexchange_1 ==
  AIB1 : Inport
  AIB2 : Inport  Port=2
  control : Inport  Port=3
  EMPTY : carnotUIBK/airexchange_intersection/EMPTY  VariantControl=(default)
  airexchange_empiric : carnotUIBK/airexchange_intersection/airexchange_empiric  VariantControl=V_i_1_2_inf1_m0
  airexchange_powerlaw : carnotUIBK/airexchange_intersection/airexchange_powerlaw  VariantControl=V_i_1_2_inf1_m1
  "[S1]" : Outport
  "[S2]" : Outport  Port=2

== system building_EXAMPLE_v2_r2018b/BUILDING/INTERSECTION_1_2/airexchange_2 ==
  AIB1 : Inport
  AIB2 : Inport  Port=2
  control : Inport  Port=3
  EMPTY : carnotUIBK/airexchange_intersection/EMPTY  VariantControl=(default)
  airexchange_empiric : carnotUIBK/airexchange_intersection/airexchange_empiric  VariantControl=V_i_1_2_inf2_m0
  airexchange_powerlaw : carnotUIBK/airexchange_intersection/airexchange_powerlaw  VariantControl=V_i_1_2_inf2_m1
  "[S1]" : Outport
  "[S2]" : Outport  Port=2

== system building_EXAMPLE_v2_r2018b/BUILDING/INTERSECTION_1_2/airexchange_3 ==
  AIB1 : Inport
  AIB2 : Inport  Port=2
  control : Inport  Port=3
  EMPTY : carnotUIBK/airexchange_intersection/EMPTY  VariantControl=(default)
  airexchange_empiric : carnotUIBK/airexchange_intersection/airexchange_empiric  VariantControl=V_i_1_2_inf3_m0
  airexchange_powerlaw : carnotUIBK/airexchange_intersection/airexchange_powerlaw  VariantControl=V_i_1_2_inf3_m1
  "[S1]" : Outport
  "[S2]" : Outport  Port=2

== system building_EXAMPLE_v2_r2018b/BUILDING/INTERSECTION_1_2/wall_1 ==
  AIB1 : Inport
  AIB2 : Inport  Port=2
  Qdot_sol1 : Inport  Port=3
  Qdot_sol2 : Inport  Port=4
  EMPTY : carnotUIBK/wall_intersection/EMPTY  VariantControl=(default)
  R-C model : carnotUIBK/wall_intersection/R-C model  VariantControl=V_i_1_2_w1_m1  t0=z.t_ini  d=fliplr(const.parameter.xmesh_beu)  cond=fliplr(const.parameter.lambda)  cwall=fliplr(const.parameter.cp)  rho=fliplr(const.parameter.rho)  reflectground=0.2  abs_emiss=[const.absorption_2 const.emission_2 const.emission_1]  tau=const.parameter.tau  dactive=const.parameter.d_active
      link override alpha_i1/alpha_i_down: VariantControl=V_i_1_2_w1_hti2
      link override alpha_i1/alpha_i_horizontal: VariantControl=V_i_1_2_w1_hti0
      link override alpha_i1/alpha_i_up: VariantControl=V_i_1_2_w1_hti1
      link override alpha_i2/alpha_i_down: VariantControl=V_i_1_2_w1_hti2
      link override alpha_i2/alpha_i_horizontal: VariantControl=V_i_1_2_w1_hti0
      link override alpha_i2/alpha_i_up: VariantControl=V_i_1_2_w1_hti1
  UA : carnotUIBK/wall_intersection/UA  VariantControl=V_i_1_2_w1_m0  U=const.parameter.U
      link override Rsi/down: VariantControl=V_i_1_2_w1_hti2
      link override Rsi/horizontal: VariantControl=V_i_1_2_w1_hti0
      link override Rsi/up: VariantControl=V_i_1_2_w1_hti1
  hygrothermal model : carnotUIBK/wall_intersection/hygrothermal model  VariantControl=V_i_1_2_w1_m2  t0=z.t_ini  reflectground=0.2  abs_emiss=[const.absorption_2 const.emission_2 const.emission_1]  xmesh=const.parameter.xmesh_hygro  X=const.parameter.X  d=const.parameter.d  lambda=const.parameter.lambda_hygro  rho=const.parameter.rho_hygro  cp=const.parameter.cp_hygro  mu=const.parameter.mu  ufs=const.parameter.ufs  FSF_u=const.parameter.FSF_u  FSF_phi=const.parameter.FSF_phi  FSF_dudphi=const.parameter.FSF_dudphi  FSF_k=const.parameter.FSF_k  K_kleff=const.parameter.K_kleff  K_u=const.parameter.K_u  K_kl=const.parameter.K_kl  FSF_length=const.parameter.FSF_length  K_length=const.parameter.K_length  T_ini=const.parameter.T_ini_hygro  Phi_ini=const.parameter.Phi_ini_hygro  T_source=const.parameter.T_source  Phi_source=const.parameter.Phi_source  Tdactive=const.parameter.T_dactive  Phidactive=const.parameter.Phi_dactive
      link override alpha_i1/alpha_i_down: VariantControl=V_i_1_2_w1_hti2
      link override alpha_i1/alpha_i_horizontal: VariantControl=V_i_1_2_w1_hti0
      link override alpha_i1/alpha_i_up: VariantControl=V_i_1_2_w1_hti1
      link override alpha_i2/alpha_i_down: VariantControl=V_i_1_2_w1_hti2
      link override alpha_i2/alpha_i_horizontal: VariantControl=V_i_1_2_w1_hti0
      link override alpha_i2/alpha_i_up: VariantControl=V_i_1_2_w1_hti1
  "[S1]" : Outport
  "[S2]" : Outport  Port=2

== system building_EXAMPLE_v2_r2018b/BUILDING/INTERSECTION_1_2/wall_2 ==
  AIB1 : Inport
  AIB2 : Inport  Port=2
  Qdot_sol1 : Inport  Port=3
  Qdot_sol2 : Inport  Port=4
  EMPTY : carnotUIBK/wall_intersection/EMPTY  VariantControl=(default)
  R-C model : carnotUIBK/wall_intersection/R-C model  VariantControl=V_i_1_2_w2_m1  t0=z.t_ini  d=fliplr(const.parameter.xmesh_beu)  cond=fliplr(const.parameter.lambda)  cwall=fliplr(const.parameter.cp)  rho=fliplr(const.parameter.rho)  reflectground=0.2  abs_emiss=[const.absorption_2 const.emission_2 const.emission_1]  tau=const.parameter.tau  dactive=const.parameter.d_active
      link override alpha_i1/alpha_i_down: VariantControl=V_i_1_2_w2_hti2
      link override alpha_i1/alpha_i_horizontal: VariantControl=V_i_1_2_w2_hti0
      link override alpha_i1/alpha_i_up: VariantControl=V_i_1_2_w2_hti1
      link override alpha_i2/alpha_i_down: VariantControl=V_i_1_2_w2_hti2
      link override alpha_i2/alpha_i_horizontal: VariantControl=V_i_1_2_w2_hti0
      link override alpha_i2/alpha_i_up: VariantControl=V_i_1_2_w2_hti1
  UA : carnotUIBK/wall_intersection/UA  VariantControl=V_i_1_2_w2_m0  U=const.parameter.U
      link override Rsi/down: VariantControl=V_i_1_2_w2_hti2
      link override Rsi/horizontal: VariantControl=V_i_1_2_w2_hti0
      link override Rsi/up: VariantControl=V_i_1_2_w2_hti1
  hygrothermal model : carnotUIBK/wall_intersection/hygrothermal model  VariantControl=V_i_1_2_w2_m2  t0=z.t_ini  reflectground=0.2  abs_emiss=[const.absorption_2 const.emission_2 const.emission_1]  xmesh=const.parameter.xmesh_hygro  X=const.parameter.X  d=const.parameter.d  lambda=const.parameter.lambda_hygro  rho=const.parameter.rho_hygro  cp=const.parameter.cp_hygro  mu=const.parameter.mu  ufs=const.parameter.ufs  FSF_u=const.parameter.FSF_u  FSF_phi=const.parameter.FSF_phi  FSF_dudphi=const.parameter.FSF_dudphi  FSF_k=const.parameter.FSF_k  K_kleff=const.parameter.K_kleff  K_u=const.parameter.K_u  K_kl=const.parameter.K_kl  FSF_length=const.parameter.FSF_length  K_length=const.parameter.K_length  T_ini=const.parameter.T_ini_hygro  Phi_ini=const.parameter.Phi_ini_hygro  T_source=const.parameter.T_source  Phi_source=const.parameter.Phi_source  Tdactive=const.parameter.T_dactive  Phidactive=const.parameter.Phi_dactive
      link override alpha_i1/alpha_i_down: VariantControl=V_i_1_2_w2_hti2
      link override alpha_i1/alpha_i_horizontal: VariantControl=V_i_1_2_w2_hti0
      link override alpha_i1/alpha_i_up: VariantControl=V_i_1_2_w2_hti1
      link override alpha_i2/alpha_i_down: VariantControl=V_i_1_2_w2_hti2
      link override alpha_i2/alpha_i_horizontal: VariantControl=V_i_1_2_w2_hti0
      link override alpha_i2/alpha_i_up: VariantControl=V_i_1_2_w2_hti1
  "[S1]" : Outport
  "[S2]" : Outport  Port=2

== system building_EXAMPLE_v2_r2018b/BUILDING/INTERSECTION_1_2/wall_3 ==
  AIB1 : Inport
  AIB2 : Inport  Port=2
  Qdot_sol1 : Inport  Port=3
  Qdot_sol2 : Inport  Port=4
  EMPTY : carnotUIBK/wall_intersection/EMPTY  VariantControl=(default)
  R-C model : carnotUIBK/wall_intersection/R-C model  VariantControl=V_i_1_2_w3_m1  t0=z.t_ini  d=fliplr(const.parameter.xmesh_beu)  cond=fliplr(const.parameter.lambda)  cwall=fliplr(const.parameter.cp)  rho=fliplr(const.parameter.rho)  reflectground=0.2  abs_emiss=[const.absorption_2 const.emission_2 const.emission_1]  tau=const.parameter.tau  dactive=const.parameter.d_active
      link override alpha_i1/alpha_i_down: VariantControl=V_i_1_2_w3_hti2
      link override alpha_i1/alpha_i_horizontal: VariantControl=V_i_1_2_w3_hti0
      link override alpha_i1/alpha_i_up: VariantControl=V_i_1_2_w3_hti1
      link override alpha_i2/alpha_i_down: VariantControl=V_i_1_2_w3_hti2
      link override alpha_i2/alpha_i_horizontal: VariantControl=V_i_1_2_w3_hti0
      link override alpha_i2/alpha_i_up: VariantControl=V_i_1_2_w3_hti1
  UA : carnotUIBK/wall_intersection/UA  VariantControl=V_i_1_2_w3_m0  U=const.parameter.U
      link override Rsi/down: VariantControl=V_i_1_2_w3_hti2
      link override Rsi/horizontal: VariantControl=V_i_1_2_w3_hti0
      link override Rsi/up: VariantControl=V_i_1_2_w3_hti1
  hygrothermal model : carnotUIBK/wall_intersection/hygrothermal model  VariantControl=V_i_1_2_w3_m2  t0=z.t_ini  reflectground=0.2  abs_emiss=[const.absorption_2 const.emission_2 const.emission_1]  xmesh=const.parameter.xmesh_hygro  X=const.parameter.X  d=const.parameter.d  lambda=const.parameter.lambda_hygro  rho=const.parameter.rho_hygro  cp=const.parameter.cp_hygro  mu=const.parameter.mu  ufs=const.parameter.ufs  FSF_u=const.parameter.FSF_u  FSF_phi=const.parameter.FSF_phi  FSF_dudphi=const.parameter.FSF_dudphi  FSF_k=const.parameter.FSF_k  K_kleff=const.parameter.K_kleff  K_u=const.parameter.K_u  K_kl=const.parameter.K_kl  FSF_length=const.parameter.FSF_length  K_length=const.parameter.K_length  T_ini=const.parameter.T_ini_hygro  Phi_ini=const.parameter.Phi_ini_hygro  T_source=const.parameter.T_source  Phi_source=const.parameter.Phi_source  Tdactive=const.parameter.T_dactive  Phidactive=const.parameter.Phi_dactive
      link override alpha_i1/alpha_i_down: VariantControl=V_i_1_2_w3_hti2
      link override alpha_i1/alpha_i_horizontal: VariantControl=V_i_1_2_w3_hti0
      link override alpha_i1/alpha_i_up: VariantControl=V_i_1_2_w3_hti1
      link override alpha_i2/alpha_i_down: VariantControl=V_i_1_2_w3_hti2
      link override alpha_i2/alpha_i_horizontal: VariantControl=V_i_1_2_w3_hti0
      link override alpha_i2/alpha_i_up: VariantControl=V_i_1_2_w3_hti1
  "[S1]" : Outport
  "[S2]" : Outport  Port=2

== system building_EXAMPLE_v2_r2018b/BUILDING/INTERSECTION_1_3/airexchange_1 ==
  AIB1 : Inport
  AIB2 : Inport  Port=2
  control : Inport  Port=3
  EMPTY : carnotUIBK/airexchange_intersection/EMPTY  VariantControl=(default)
  airexchange_empiric : carnotUIBK/airexchange_intersection/airexchange_empiric  VariantControl=V_i_1_3_inf1_m0
  airexchange_powerlaw : carnotUIBK/airexchange_intersection/airexchange_powerlaw  VariantControl=V_i_1_3_inf1_m1
  "[S1]" : Outport
  "[S2]" : Outport  Port=2

== system building_EXAMPLE_v2_r2018b/BUILDING/INTERSECTION_1_3/airexchange_2 ==
  AIB1 : Inport
  AIB2 : Inport  Port=2
  control : Inport  Port=3
  EMPTY : carnotUIBK/airexchange_intersection/EMPTY  VariantControl=(default)
  airexchange_empiric : carnotUIBK/airexchange_intersection/airexchange_empiric  VariantControl=V_i_1_3_inf2_m0
  airexchange_powerlaw : carnotUIBK/airexchange_intersection/airexchange_powerlaw  VariantControl=V_i_1_3_inf2_m1
  "[S1]" : Outport
  "[S2]" : Outport  Port=2

== system building_EXAMPLE_v2_r2018b/BUILDING/INTERSECTION_1_3/airexchange_3 ==
  AIB1 : Inport
  AIB2 : Inport  Port=2
  control : Inport  Port=3
  EMPTY : carnotUIBK/airexchange_intersection/EMPTY  VariantControl=(default)
  airexchange_empiric : carnotUIBK/airexchange_intersection/airexchange_empiric  VariantControl=V_i_1_3_inf3_m0
  airexchange_powerlaw : carnotUIBK/airexchange_intersection/airexchange_powerlaw  VariantControl=V_i_1_3_inf3_m1
  "[S1]" : Outport
  "[S2]" : Outport  Port=2

== system building_EXAMPLE_v2_r2018b/BUILDING/INTERSECTION_1_3/wall_1 ==
  AIB1 : Inport
  AIB2 : Inport  Port=2
  Qdot_sol1 : Inport  Port=3
  Qdot_sol2 : Inport  Port=4
  EMPTY : carnotUIBK/wall_intersection/EMPTY  VariantControl=(default)
  R-C model : carnotUIBK/wall_intersection/R-C model  VariantControl=V_i_1_3_w1_m1  t0=z.t_ini  d=fliplr(const.parameter.xmesh_beu)  cond=fliplr(const.parameter.lambda)  cwall=fliplr(const.parameter.cp)  rho=fliplr(const.parameter.rho)  reflectground=0.2  abs_emiss=[const.absorption_2 const.emission_2 const.emission_1]  tau=const.parameter.tau  dactive=const.parameter.d_active
      link override alpha_i1/alpha_i_down: VariantControl=V_i_1_3_w1_hti2
      link override alpha_i1/alpha_i_horizontal: VariantControl=V_i_1_3_w1_hti0
      link override alpha_i1/alpha_i_up: VariantControl=V_i_1_3_w1_hti1
      link override alpha_i2/alpha_i_down: VariantControl=V_i_1_3_w1_hti2
      link override alpha_i2/alpha_i_horizontal: VariantControl=V_i_1_3_w1_hti0
      link override alpha_i2/alpha_i_up: VariantControl=V_i_1_3_w1_hti1
  UA : carnotUIBK/wall_intersection/UA  VariantControl=V_i_1_3_w1_m0  U=const.parameter.U
      link override Rsi/down: VariantControl=V_i_1_3_w1_hti2
      link override Rsi/horizontal: VariantControl=V_i_1_3_w1_hti0
      link override Rsi/up: VariantControl=V_i_1_3_w1_hti1
  hygrothermal model : carnotUIBK/wall_intersection/hygrothermal model  VariantControl=V_i_1_3_w1_m2  t0=z.t_ini  reflectground=0.2  abs_emiss=[const.absorption_2 const.emission_2 const.emission_1]  xmesh=const.parameter.xmesh_hygro  X=const.parameter.X  d=const.parameter.d  lambda=const.parameter.lambda_hygro  rho=const.parameter.rho_hygro  cp=const.parameter.cp_hygro  mu=const.parameter.mu  ufs=const.parameter.ufs  FSF_u=const.parameter.FSF_u  FSF_phi=const.parameter.FSF_phi  FSF_dudphi=const.parameter.FSF_dudphi  FSF_k=const.parameter.FSF_k  K_kleff=const.parameter.K_kleff  K_u=const.parameter.K_u  K_kl=const.parameter.K_kl  FSF_length=const.parameter.FSF_length  K_length=const.parameter.K_length  T_ini=const.parameter.T_ini_hygro  Phi_ini=const.parameter.Phi_ini_hygro  T_source=const.parameter.T_source  Phi_source=const.parameter.Phi_source  Tdactive=const.parameter.T_dactive  Phidactive=const.parameter.Phi_dactive
      link override alpha_i1/alpha_i_down: VariantControl=V_i_1_3_w1_hti2
      link override alpha_i1/alpha_i_horizontal: VariantControl=V_i_1_3_w1_hti0
      link override alpha_i1/alpha_i_up: VariantControl=V_i_1_3_w1_hti1
      link override alpha_i2/alpha_i_down: VariantControl=V_i_1_3_w1_hti2
      link override alpha_i2/alpha_i_horizontal: VariantControl=V_i_1_3_w1_hti0
      link override alpha_i2/alpha_i_up: VariantControl=V_i_1_3_w1_hti1
  "[S1]" : Outport
  "[S2]" : Outport  Port=2

== system building_EXAMPLE_v2_r2018b/BUILDING/INTERSECTION_1_3/wall_2 ==
  AIB1 : Inport
  AIB2 : Inport  Port=2
  Qdot_sol1 : Inport  Port=3
  Qdot_sol2 : Inport  Port=4
  EMPTY : carnotUIBK/wall_intersection/EMPTY  VariantControl=(default)
  R-C model : carnotUIBK/wall_intersection/R-C model  VariantControl=V_i_1_3_w2_m1  t0=z.t_ini  d=fliplr(const.parameter.xmesh_beu)  cond=fliplr(const.parameter.lambda)  cwall=fliplr(const.parameter.cp)  rho=fliplr(const.parameter.rho)  reflectground=0.2  abs_emiss=[const.absorption_2 const.emission_2 const.emission_1]  tau=const.parameter.tau  dactive=const.parameter.d_active
      link override alpha_i1/alpha_i_down: VariantControl=V_i_1_3_w2_hti2
      link override alpha_i1/alpha_i_horizontal: VariantControl=V_i_1_3_w2_hti0
      link override alpha_i1/alpha_i_up: VariantControl=V_i_1_3_w2_hti1
      link override alpha_i2/alpha_i_down: VariantControl=V_i_1_3_w2_hti2
      link override alpha_i2/alpha_i_horizontal: VariantControl=V_i_1_3_w2_hti0
      link override alpha_i2/alpha_i_up: VariantControl=V_i_1_3_w2_hti1
  UA : carnotUIBK/wall_intersection/UA  VariantControl=V_i_1_3_w2_m0  U=const.parameter.U
      link override Rsi/down: VariantControl=V_i_1_3_w2_hti2
      link override Rsi/horizontal: VariantControl=V_i_1_3_w2_hti0
      link override Rsi/up: VariantControl=V_i_1_3_w2_hti1
  hygrothermal model : carnotUIBK/wall_intersection/hygrothermal model  VariantControl=V_i_1_3_w2_m2  t0=z.t_ini  reflectground=0.2  abs_emiss=[const.absorption_2 const.emission_2 const.emission_1]  xmesh=const.parameter.xmesh_hygro  X=const.parameter.X  d=const.parameter.d  lambda=const.parameter.lambda_hygro  rho=const.parameter.rho_hygro  cp=const.parameter.cp_hygro  mu=const.parameter.mu  ufs=const.parameter.ufs  FSF_u=const.parameter.FSF_u  FSF_phi=const.parameter.FSF_phi  FSF_dudphi=const.parameter.FSF_dudphi  FSF_k=const.parameter.FSF_k  K_kleff=const.parameter.K_kleff  K_u=const.parameter.K_u  K_kl=const.parameter.K_kl  FSF_length=const.parameter.FSF_length  K_length=const.parameter.K_length  T_ini=const.parameter.T_ini_hygro  Phi_ini=const.parameter.Phi_ini_hygro  T_source=const.parameter.T_source  Phi_source=const.parameter.Phi_source  Tdactive=const.parameter.T_dactive  Phidactive=const.parameter.Phi_dactive
      link override alpha_i1/alpha_i_down: VariantControl=V_i_1_3_w2_hti2
      link override alpha_i1/alpha_i_horizontal: VariantControl=V_i_1_3_w2_hti0
      link override alpha_i1/alpha_i_up: VariantControl=V_i_1_3_w2_hti1
      link override alpha_i2/alpha_i_down: VariantControl=V_i_1_3_w2_hti2
      link override alpha_i2/alpha_i_horizontal: VariantControl=V_i_1_3_w2_hti0
      link override alpha_i2/alpha_i_up: VariantControl=V_i_1_3_w2_hti1
  "[S1]" : Outport
  "[S2]" : Outport  Port=2
